simulink model "Es2_1slx"  (R2014a)
settings: Solver=ode45  StartTime=0.0  StopTime=10.0  RelTol=1e-3
values from neighbouring files (symbols this model uses):
  F1 = (Ka*Km)/(s^2*J*La + s*(Beta*La + J*Ra) + Beta*Ra + Km^2)    [Es1_1.m]    (also in Es1_2.m; Es2_1.m; Es2_2.m)
  F2 = -(s*La + Ra)/(s^2*J*La + s*(Beta*La + J*Ra) + Beta*Ra + Km^2)    [Es1_1.m]    (also in Es1_2.m; Es2_1.m; Es2_2.m)
  s = tf('s')    [Es1_1.m]    (also in Es1_2.m; Es2_1.m; Es2_2.m)
libraries: cstblocks x2
settings Model: Creator=UTENTE  LastModifiedBy=UTENTE

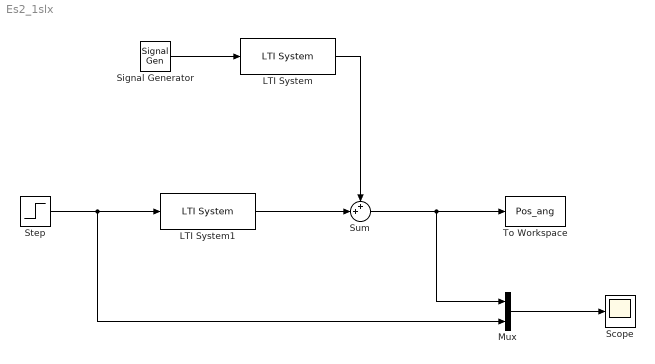
== system Es2_1slx ==
  LTI System : cstblocks/LTI System  sys=F2/s  IC=[]
  LTI System1 : cstblocks/LTI System  sys=F1/s  IC=[]
  Mux : Mux  Inputs=2
  Scope : Scope
  Signal Generator : SignalGenerator  WaveForm=square  Amplitude=0.05  Frequency=0.1
  Step : Step  Time=0  SampleTime=0
  Sum : Sum  Inputs=++|
  To Workspace : ToWorkspace  VariableName=Pos_ang  SaveFormat=Timeseries  SampleTime=-1
  wires:
  Signal Generator/1 -> LTI System/1
  Step/1 -> Mux/2, LTI System1/1
  LTI System/1 -> Sum/1
  LTI System1/1 -> Sum/2
  Sum/1 -> Mux/1, To Workspace/1
  Mux/1 -> Scope/1
